simulink model "TPTC_Vehicle_dynamics_pedal2torque_NeglectSOC"  (R2026a)
settings: Solver=ode23tb  StopTime=40
model workspace (MAT data in the model file):
  BattChrgMax = -500000
  BattDischrgMax = 500000
  ChrgLmt_bpt = [1 1 1 1 1 1 1 1 0.7 0.35 0]
  DischrgLmt_bpt = [0 0.35 0.7 1 1 1 1 1 1 1 1]
  SOC_bpt = [0 10 20 30 40 50 60 70 80 90 100]
  motorMaxTorqueNm = [500 500 500 500 500 500 416.666666667 357.142857143 312.5 277.777777778 250 227.272727273 208.333333333 192.307692308 178.571428571 166.666666667]
  motorSpeedRadPs = [0 40 80 120 160 200 240 280 320 360 400 440 480 520 560 600]
values from neighbouring files (symbols this model uses):
  alpha_thr = Simulink.Parameter(300)    [init_MCU_ASR_params_only.m]
  eta_drv = Simulink.Parameter(0.95)    [init_MCU_ASR_params_only.m]
  gear_ratio_F = Simulink.Parameter(10.91)    [init_MCU_ASR_params_only.m]
  gear_ratio_R = Simulink.Parameter(11.62)    [init_MCU_ASR_params_only.m]
  J_axle = Simulink.Parameter(2*I_tire)    [init_MCU_ASR_params_only.m]
  Kd_damp = Simulink.Parameter(0.025)    [init_MCU_ASR_params_only.m]
  R_tire = Simulink.Parameter(r)    [init_MCU_ASR_params_only.m]
  T_active = Simulink.Parameter(15)    [init_MCU_ASR_params_only.m]
  T_damp_lim = Simulink.Parameter(18)    [init_MCU_ASR_params_only.m]
  tau_lpf_damp = Simulink.Parameter(0.060)    [init_MCU_ASR_params_only.m]
  Tlim_down_rate = Simulink.Parameter(2000)    [init_MCU_ASR_params_only.m]
  Tlim_up_rate = Simulink.Parameter(120)    [init_MCU_ASR_params_only.m]
  Tlim_warn_rate = Simulink.Parameter(600)    [init_MCU_ASR_params_only.m]
  Tmax_mot = Simulink.Parameter(Tn_motor)    [init_MCU_ASR_params_only.m]
  Ts_asr = Simulink.Parameter(0.001)    [init_MCU_ASR_params_only.m]
undefined symbols (not defined in the file or in its folder): dspblkCoreblockFVToolHelper, gcbh, gear_ratio
libraries: autolibsharedcoupling x8, simulink x3, autolibshareddiff x2, autolibmappedmotor x2, slpidlib x1, autolibdatasheetbattery x1, sim3dlib x1, sim3dautolib x1, vehdynlibsteering x1
(part 1 of 4)
settings Model: Creator=jchu  LastModifiedBy=woaiw

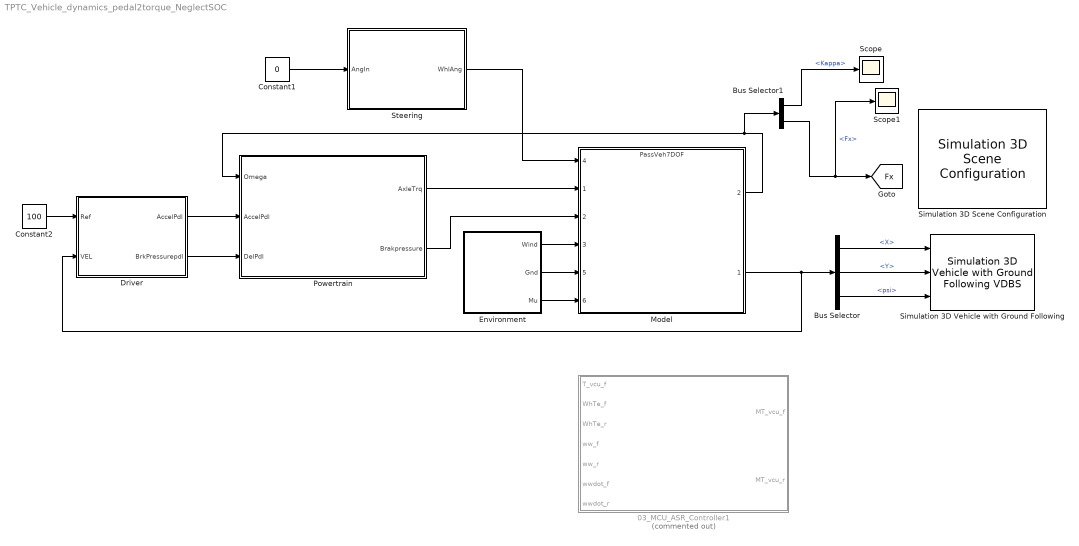
== system TPTC_Vehicle_dynamics_pedal2torque_NeglectSOC ==
  03_MCU_ASR_Controller1 : Subsystem  Commented=on
  Bus Selector : BusSelector  OutputSignals=InertFrm.Cg.Disp.X,InertFrm.Cg.Disp.Y,InertFrm.Cg.Ang.psi
  Bus Selector1 : BusSelector  OutputSignals=TireFrame.Kappa,TireFrame.Fx
  Constant1 : Constant  Value=0
  Constant2 : Constant  Value=100
  Driver : Subsystem
  Environment : Subsystem
      mask Display: disp('Environment')
  Model : ModelReference  ModelNameDialog=PassVeh7DOF.slx  SimulationMode=Normal  ModelReferenceVersion=9.3
      settings: PortSchema="{\"entries\":[{\"content\":{\"sides\":[{\"content\":{\"connectorIds\":[\"In4\",\"In1\",\"In2\",\"In3\",\"In5\",\"In6\"]},\"type\":\"ConnectorPlacement.EquallySpacedRectSide\",\"uuid\":\"e9709a47-3cb3-4a3a-94dc-e137fda36ac7\"},{\"content\":{\"connectorIds\":[\"Out2\",\"Out1\"],\"side\":\"RIGHT\"},\"type\":\"ConnectorPlacement.EquallySpacedRectSide\",\"uuid\":\"17c9465a-c7d2-47f9-932e-b722968c60f5\"},{\"content\":{\"side\":\"TOP\"},\"type\":\"ConnectorPlacement.EquallySpacedRectSide\",\"uuid\":\"38cd0d31-1510-4d7f-a224-4b6e7eb516ec\"}]},\"type\":\"ConnectorPlacement.EquallySpacedConnector\",\"uuid\":\"ef4f9ae8-cb52-4422-b25b-7a352d7601ce\"}],\"packageUris\":[\"http://schema.mathworks.com/mf0/Connector/R2020b\"],\"version\":\"1.0\"}"
  Powertrain : Subsystem
      mask DialogControl ParameterGroupVar Prompt: 参数
      mask Display: image('vdbslibpt.png');
  Scope : Scope
      settings: ActiveDisplayYMinimum=-0.1162629811847193  ActiveDisplayYMaximum=1.0459974821651312  DataLoggingVariableName=ScopeData10
  Scope1 : Scope
      settings: ActiveDisplayYMinimum=-501.51287  ActiveDisplayYMaximum=4500.86669  DataLoggingVariableName=ScopeData9
  Simulation 3D Scene Configuration : sim3dlib/Simulation 3D Scene Configuration  Priority=0  ProjectFormat=Default Scenes  SceneDesc=Straight road  ProjectName=D:\Program Files\MATLAB\R2026a\toolbox\shared\sim3d_projects\automotive_project_windows\UE\WindowsNoEditor\VehicleSimulation.exe  ScenePath=/Game/Maps/HwStrght  EnableOpenDRIVE=off  vehTagList={'Custom';'Scene Origin';'SimulinkVehicle1'}  vehTag=SimulinkVehicle1  AttachedCameraRelativeTranslation=[0 0 0]  FreeCameraDefaultInitialTranslation=[-6, 0, 2]  AttachedCameraRelativeRotation=[0, -15, 0]  FreeCameraDefaultInitialRotation=[0, -15, 0]  ViewpointName=Custom  FreeCameraInitialTranslation=[0, 0, 0]  FreeCameraInitialRotation=[0, 0, 0]  OpVisEn=off  Ts=.02  EnableWindow=on  EnableRemoteAccess=off  SimulationMode=CoSimulation  SimulateUsing=Interpreted execution  EnableAnimationRecording=off  OverrideDefaultRecording=off  AnimationRecordingFileName=sim3dAnimation.mat  AnimationRecordingInterval=[0 inf]  EnableWeather=off  SunAzimuth=90  SunAltitude=40.0  EnableGeospatialSun=off  Latitude=0  Longitude=0  Date=2023-01-01  Time=10:30:00  GeoTimeZone=-5.0  SunDaylightSaving=off  wind=1  clouds=10  EnableVolumetricClouds=off  CloudCoverage=0  CloudAltitude=6  fog=0  rain=0  RaindropsEffect=off  SnowDensity=0  EnableGeospatial=off  TilesetSource=Earth terrain  UseTrueOrigin=off  OriginHeight=200  OriginLatitude=40.744652  OriginLongitude=-73.988864  MapStyle=Aerial  AdditionalAssetIDs=[]  UseAdvancedSunSky=off  SolarTime=11  TimeZone=-5  Day=21  Month=9  Year=2022  UseDaylightSavingTime=on  DSTStartDay=10  DSTStartMonth=3  DSTEndDay=3  DSTEndMonth=11  DSTSwitchHour=2  sensorTag=MainCamera1  sensorId=1  sensorName=MainCamera1  mountLoc=Origin  offsetFlag=off  tmountOffset=[0, 0, 0]  rmountOffset=[0, 0, 0]  HorizontalResolution=1280  VerticalResolution=720  HorizontalFOV=60  mountPoint=[0 0 0]  mountOrientation=[0 0 0]  aMode=2  ID=1  GeoTrigger=Inactive  ViewNameList={'Custom'}  ViewTranslationList={'[0 0 0]'}  ViewRotationList={'[0 0 0]'}
      settings: LibrarySourceBlock=vehdynlibsim3dcore/Simulation 3D Scene Configuration
  Simulation 3D Vehicle with Ground Following : sim3dautolib/Simulation 3D Vehicle with Ground Following VDBS  Priority=-1  PassVehMesh=Muscle car  MeshPath=/MathWorksSimulation/Vehicles/Muscle/Meshes/SK_MuscleCar.SK_MuscleCar  TrackWidth=1.9  WheelBase=3  WheelRadius=0.35  VehColor=Red  CoordinateSystem=Default  InitialPos=[0, 0, 0]  InitialRot=[0, 0, 0]  ActorName=SimulinkVehicle1  VehLightsControl=off  HeadlightColor=[ 1, 1, 1 ]  HighBeamIntensity=100000  LowBeamIntensity=60000  HighBeamConeAngle=1.22  LowBeamConeAngle=1.22  LeftHeadlightOrientation=[ 0, 0 ]  RightHeadlightOrientation=[ 0, 0 ]  BrakelightIntensity=200  ReverselightIntensity=500  SignallightIntensity=500  SignallightPeriod=1  SignalPulseWidth=50  SampleTime=-1  ActorType=SimulinkVehicle  ID=1  aMode=2  ActorTag=SimulinkVehicle1  CoordinateScheme=SAE
      settings: LibrarySourceBlock=vehdynlibsim3d/Simulation 3D Vehicle with Ground Following
  Steering : Subsystem
  tag scope: Fx=global
  wires:
  Bus Selector/2 -> Simulation 3D Vehicle with Ground Following/2  "<Y>"
  Bus Selector/1 -> Simulation 3D Vehicle with Ground Following/1  "<X>"
  Bus Selector/3 -> Simulation 3D Vehicle with Ground Following/3  "<psi>"
  Environment/1(Wind) -> Model/3
  Environment/2(Gnd) -> Model/5
  Environment/3(Mu) -> Model/6
  Constant1/1 -> Steering/1(AngIn)
  Steering/1(WhlAng) -> Model/4
  Model/2 -> Bus Selector1/1, Powertrain/1(Omega)
  Powertrain/2(Brakpressure) -> Model/2
  Constant2/1 -> Driver/1(Ref)
  Model/1 -> Driver/2(VEL), Bus Selector/1
  Driver/1(AccelPdl) -> Powertrain/2(AccelPdl)
  Driver/2(BrkPressurepdl) -> Powertrain/3(DelPdl)
  Powertrain/1(AxleTrq) -> Model/1
  Bus Selector1/1 -> Scope/1  "<Kappa>"
  Bus Selector1/2 -> Scope1/1, [Fx]  "<Fx>"

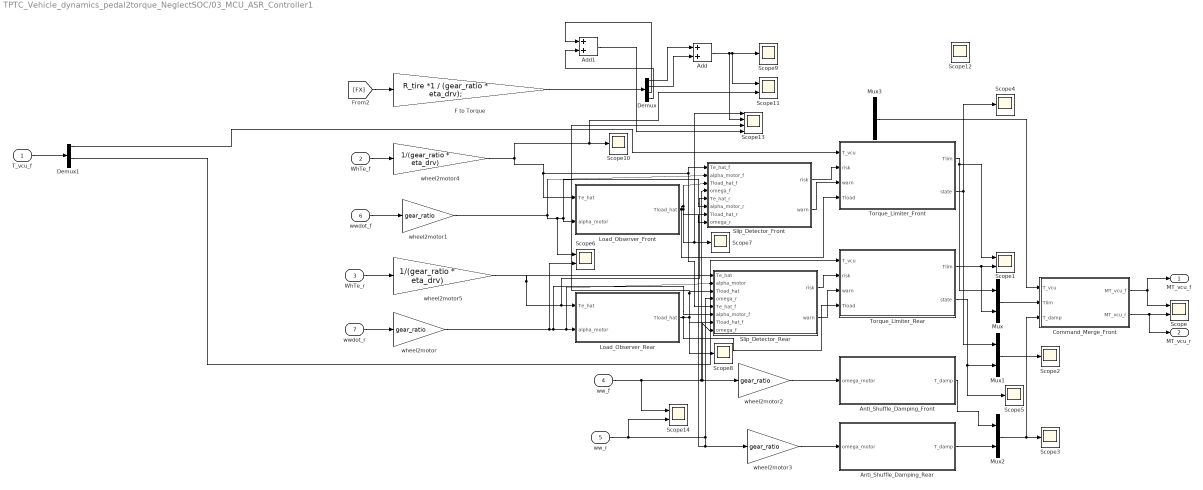
== system TPTC_Vehicle_dynamics_pedal2torque_NeglectSOC/03_MCU_ASR_Controller1 ==
  T_vcu_f : Inport
  WhTe_f : Inport  Port=2
  WhTe_r : Inport  Port=3
  ww_f : Inport  Port=4
  ww_r : Inport  Port=5
  wwdot_f : Inport  Port=6
  wwdot_r : Inport  Port=7
  Add : Sum
  Add1 : Sum
  Anti_Shuffle_Damping_Front : Subsystem
  Anti_Shuffle_Damping_Rear : Subsystem
  Command_Merge_Front : Subsystem
  Demux : Demux
  Demux1 : Demux
  F to Torque : Gain  Gain=R_tire *1 / (gear_ratio * eta_drv);
  Load_Observer_Front : Subsystem
  Load_Observer_Rear : Subsystem
  Mux{,1..3} (4 alike) : Mux  Inputs=2
  Scope{,1,6,11..12,14} (6 alike) : Scope  NumInputPorts=2
      Scope settings: ActiveDisplayYMinimum=-22.2669  ActiveDisplayYMaximum=200.40213  DataLoggingVariableName=ScopeData4
      Scope1 settings: ActiveDisplayYMinimum=-22.33565  ActiveDisplayYMaximum=201.02089  DataLoggingVariableName=ScopeData7
      Scope11 settings: ActiveDisplayYMinimum=-46.74618  ActiveDisplayYMaximum=367.09259  DataLoggingVariableName=ScopeData15
      Scope12 settings: ActiveDisplayYMinimum=-100  ActiveDisplayYMaximum=900  DataLoggingVariableName=ScopeData18
      Scope14 settings: ActiveDisplayYMinimum=23.34376  ActiveDisplayYMaximum=406.47833
      Scope6 settings: ActiveDisplayYMinimum=-2816.65932  ActiveDisplayYMaximum=2610.1461  DataLoggingVariableName=ScopeData11
  Scope{2..5,7..10} (8 alike) : Scope
      Scope10 settings: ActiveDisplayYMinimum=-31.66736  ActiveDisplayYMaximum=285.00624  DataLoggingVariableName=ScopeData12
      Scope2 settings: ActiveDisplayYMinimum=-0.5  ActiveDisplayYMaximum=4.5
      Scope3 settings: ActiveDisplayYMinimum=-15.80377  ActiveDisplayYMaximum=2.40338  DataLoggingVariableName=ScopeData8
      Scope4 settings: ActiveDisplayYMinimum=-0.5  ActiveDisplayYMaximum=4.5  DataLoggingVariableName=ScopeData9
      Scope5 settings: ActiveDisplayYMinimum=-0.5  ActiveDisplayYMaximum=4.5  DataLoggingVariableName=ScopeData10
      Scope7 settings: ActiveDisplayYMinimum=-37.43965  ActiveDisplayYMaximum=336.95687  DataLoggingVariableName=ScopeData4
      Scope8 settings: ActiveDisplayYMinimum=-35.86607  ActiveDisplayYMaximum=322.79459  DataLoggingVariableName=ScopeData5
      Scope9 settings: ActiveDisplayYMinimum=-46.74618  ActiveDisplayYMaximum=367.09259  DataLoggingVariableName=ScopeData6
  Scope13 : Scope  NumInputPorts=4
      settings: ActiveDisplayYMinimum=-50.79662  ActiveDisplayYMaximum=367.54264
  Slip_Detector_Front : Subsystem
  Slip_Detector_Rear : Subsystem
  Torque_Limiter_Front : Subsystem
  Torque_Limiter_Rear : Subsystem
  wheel2motor{,1..3} (4 alike) : Gain  Gain=gear_ratio
  wheel2motor4 : Gain  Gain=1/(gear_ratio * eta_drv)
  wheel2motor5 : Gain  Gain=1/(gear_ratio * eta_drv)
  MT_vcu_f : Outport
  MT_vcu_r : Outport  Port=2
  wires:
  wwdot_f/1 -> wheel2motor1/1
  wwdot_r/1 -> wheel2motor/1
  Load_Observer_Rear/1(Tload_hat) -> Torque_Limiter_Rear/4(Tload), Scope13/3, Slip_Detector_Rear/3(Tload_hat), Scope8/1, Slip_Detector_Rear/7(Tload_hat_f)
  WhTe_r/1 -> wheel2motor5/1
  WhTe_f/1 -> wheel2motor4/1
  wheel2motor/1 -> Slip_Detector_Rear/6(alpha_motor_f), Slip_Detector_Rear/2(alpha_motor), Load_Observer_Rear/2(alpha_motor), Scope6/2
  wheel2motor1/1 -> Scope6/1, Slip_Detector_Front/6(alpha_motor_r), Load_Observer_Front/2(alpha_motor), Slip_Detector_Front/2(alpha_motor_f)
  ww_f/1 -> Scope14/1, wheel2motor2/1, Slip_Detector_Rear/8(omega_f), Slip_Detector_Front/4(omega_f)
  Anti_Shuffle_Damping_Front/1(T_damp) -> Mux2/1
  Slip_Detector_Rear/2(warn) -> Torque_Limiter_Rear/3(warn)
  Slip_Detector_Rear/1(risk) -> Torque_Limiter_Rear/2(risk)
  Slip_Detector_Front/1(risk) -> Torque_Limiter_Front/2(risk)
  Slip_Detector_Front/2(warn) -> Torque_Limiter_Front/3(warn)
  wheel2motor2/1 -> Anti_Shuffle_Damping_Front/1(omega_motor)
  wheel2motor3/1 -> Anti_Shuffle_Damping_Rear/1(omega_motor)
  Mux3/1 -> Command_Merge_Front/1(T_vcu)
  Torque_Limiter_Front/1(Tlim) -> Scope1/1, Mux/1
  Torque_Limiter_Front/2(state) -> Mux1/1, Scope4/1
  Torque_Limiter_Rear/1(Tlim) -> Scope1/2, Mux/2
  Torque_Limiter_Rear/2(state) -> Scope5/1, Mux1/2
  Anti_Shuffle_Damping_Rear/1(T_damp) -> Mux2/2
  Mux/1 -> Command_Merge_Front/2(Tlim)
  Mux1/1 -> Scope2/1
  Mux2/1 -> Scope3/1, Command_Merge_Front/3(T_damp)
  Command_Merge_Front/1(MT_vcu_f) -> MT_vcu_f/1, Scope/1
  Command_Merge_Front/2(MT_vcu_r) -> Scope/2, MT_vcu_r/1
  [FX] -> F to Torque/1
  F to Torque/1 -> Demux/1
  Demux/1 -> Add/1
  Demux/2 -> Add/2
  wheel2motor4/1 -> Slip_Detector_Rear/5(Te_hat_f), Slip_Detector_Front/1(Te_hat_f), Load_Observer_Front/1(Te_hat), Scope11/2, Scope10/1
  wheel2motor5/1 -> Slip_Detector_Front/5(Te_hat_r), Load_Observer_Rear/1(Te_hat), Slip_Detector_Rear/1(Te_hat)
  Demux/3 -> Add1/1
  Demux/4 -> Add1/2
  Load_Observer_Front/1(Tload_hat) -> Scope13/1, Scope7/1, Slip_Detector_Front/7(Tload_hat_r), Slip_Detector_Front/3(Tload_hat_f), Torque_Limiter_Front/4(Tload)
  Add/1 -> Scope13/2, Scope11/1, Scope9/1
  Add1/1 -> Scope13/4
  ww_r/1 -> Scope14/2, wheel2motor3/1, Slip_Detector_Front/8(omega_r), Slip_Detector_Rear/4(omega_r)
  Demux1/1 -> Torque_Limiter_Front/1(T_vcu)
  Demux1/3 -> Torque_Limiter_Rear/1(T_vcu)
  T_vcu_f/1 -> Demux1/1

== system TPTC_Vehicle_dynamics_pedal2torque_NeglectSOC/Driver ==
  Ref : Inport
  VEL : Inport  Port=2
  APPDynamics : TransferFcn  Denominator=[0.75 1]
  Accel : Saturate  UpperLimit=100  LowerLimit=0
  Add : Sum  Inputs=+-
  Brake : Saturate  UpperLimit=0  LowerLimit=-100
  BrakeDynamics : TransferFcn  Denominator=[1 1]
  Bus Selector : BusSelector  OutputSignals=BdyFrm.Cg.Vel.xdot
  Gain : Gain  Gain=1/100
  Gain1 : Gain  Gain=1/100
  MakePositive : Abs  SaturateOnIntegerOverflow=off
  PID Controller : slpidlib/PID Controller  Controller=PI  Form=Parallel  TimeDomain=Continuous-time  UseExternalTs=off  SampleTime=-1  IntegratorMethod=Forward Euler  FilterMethod=Forward Euler  ControllerParametersSource=internal  P=20  I=1  UseKiTs=off  D=0  UseExternalDerivativeSource=off  N=100  UseFilter=on  TunerSelectOption=Transfer Function Based (PID Tuner App)  InitialConditionSource=internal  InitialConditionForIntegrator=0  InitialConditionForFilter=0  DifferentiatorICPrevScaledInput=0  ExternalReset=none  TrackingMode=off  Kt=1  LimitOutput=on  SatLimitsSource=internal  UpperSaturationLimit=100  LowerSaturationLimit=-100  LinearizeAsGain=on  AntiWindupMode=none  Kb=1  LimitIntegrator=off  UpperIntegratorSaturationLimit=inf  LowerIntegratorSaturationLimit=-inf  POutMin=[]  POutMax=[]  IOutMin=[]  IOutMax=[]  DOutMin=[]  DOutMax=[]  NOutMin=[]  NOutMax=[]  SumOutMin=[]  SumOutMax=[]  SaturationOutMin=[]  SaturationOutMax=[]  PParamMin=[]  PParamMax=[]  IParamMin=[]  IParamMax=[]  DParamMin=[]  DParamMax=[]  NParamMin=[]  NParamMax=[]  KbParamMin=[]  KbParamMax=[]  KtParamMin=[]  KtParamMax=[]  KbOutMin=[]  KbOutMax=[]  KtOutMin=[]  KtOutMax=[]  IntegratorOutMin=[]  IntegratorOutMax=[]  FilterOutMin=[]  FilterOutMax=[]  SumI1OutMin=[]  SumI1OutMax=[]  SumI2OutMin=[]  SumI2OutMax=[]  SumI3OutMin=[]  SumI3OutMax=[]  SumI4OutMin=[]  SumI4OutMax=[]  SumDOutMin=[]  SumDOutMax=[]  DifferentiatorOutMin=[]  DifferentiatorOutMax=[]  FilterDiffOutCoefMin=[]  FilterDiffOutCoefMax=[]  ReciprocalOutMin=[]  ReciprocalOutMax=[]  SumDenOutMin=[]  SumDenOutMax=[]  SumNumOutMin=[]  SumNumOutMax=[]  DivideOutMin=[]  DivideOutMax=[]  UdiffTsProdOutMin=[]  UdiffTsProdOutMax=[]  NTsProdOutMin=[]  NTsProdOutMax=[]  UintegralTsProdOutMin=[]  UintegralTsProdOutMax=[]  UngainTsProdOutMin=[]  UngainTsProdOutMax=[]  ClampingZeroOutDataTypeStr=Inherit: Inherit via back propagation  ClampingZeroOutMin=[]  ClampingZeroOutMax=[]  FilterDenConstantOutDataTypeStr=Inherit: Inherit via back propagation  FilterDenConstantOutMin=[]  FilterDenConstantOutMax=[]  PCopyOutDataTypeStr=Inherit: Inherit via back propagation  PCopyOutMin=[]  PCopyOutMax=[]  NCopyOutDataTypeStr=Inherit: Inherit via back propagation  NCopyOutMin=[]  NCopyOutMax=[]  IntegratorContinuousStateAttributes=''  IntegratorStateMustResolveToSignalObject=off  IntegratorRTWStateStorageClass=Auto  FilterContinuousStateAttributes=''  FilterStateMustResolveToSignalObject=off  FilterRTWStateStorageClass=Auto  ParallelPVariant=InternalParameters  IdealPVariant=Disabled  IVariant=InternalParameters  DVariant=Disabled  IntegratorVariant=Continuous  SatVariant=Enabled  AWVariant=Passthrough  PCopyVariant=Disabled  TRVariant=Disabled  FdbkBlocksVariant=Forward  IdealPFdbkVariant=Disabled  SatFdbkVariant=Disabled  DerivativeFilterVariant=Disabled  NVariant=Disabled  NCopyVariant=Disabled_SignalSpec  FilterICVariant=Disabled  IntegratorICVariant=InternalICs  ExternalResetVariant=Disabled  TRSumVariant=Passthrough  SumFdbkVariant=Disabled  SumVariant=Sum_PI  TsampFilterVariant=InternalTs  TsampNgainVariant=Passthrough  TsampIntegralVariant=Disabled_SignalSpec  ExternalSaturationOutDataTypeStr=Inherit: Same as second input  DerivativeSourceVariant=Disabled  PreIntVariant=InternalPreInt
  Scope : Scope
      settings: ActiveDisplayYMinimum=-10.41558  ActiveDisplayYMaximum=93.74018
  AccelPdl : Outport
  BrkPressurepdl : Outport  Port=2
  wires:
  APPDynamics/1 -> Gain/1
  PID Controller/1 -> Accel/1, Brake/1
  MakePositive/1 -> BrakeDynamics/1
  Accel/1 -> APPDynamics/1
  Add/1 -> PID Controller/1
  Brake/1 -> MakePositive/1
  Ref/1 -> Add/1
  BrakeDynamics/1 -> Gain1/1
  Gain/1 -> AccelPdl/1
  Gain1/1 -> BrkPressurepdl/1
  VEL/1 -> Bus Selector/1
  Bus Selector/1 -> Scope/1, Add/2  "<xdot>"

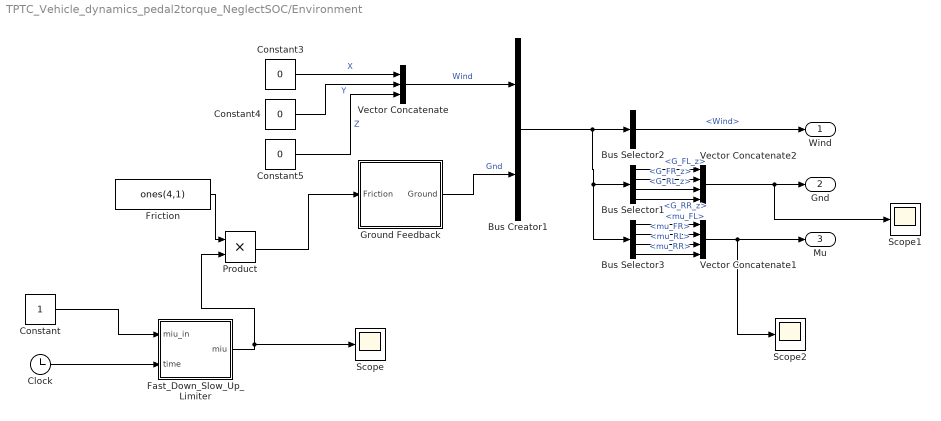
== system TPTC_Vehicle_dynamics_pedal2torque_NeglectSOC/Environment ==
  Bus Creator1 : BusCreator  Inputs=2
  Bus Selector1 : BusSelector  OutputSignals=Gnd.z.G_FL_z,Gnd.z.G_FR_z,Gnd.z.G_RL_z,Gnd.z.G_RR_z
  Bus Selector2 : BusSelector  OutputSignals=Wind
  Bus Selector3 : BusSelector  OutputSignals=Gnd.mu.mu_FL,Gnd.mu.mu_FR,Gnd.mu.mu_RL,Gnd.mu.mu_RR
  Clock : Clock
  Constant : Constant
  Constant3 : Constant  Value=0
  Constant4 : Constant  Value=0
  Constant5 : Constant  Value=0
  Fast_Down_Slow_Up_Limiter : MATLAB Function  TreatAsAtomicUnit=on  SystemSampleTime=Ts_asr
  Friction : Constant  Value=ones(4,1)
  Ground Feedback : Subsystem  Variant=on  VariantControlMode=label  LabelModeActiveChoice=0
  Product : Product
  Scope : Scope
      settings: ActiveDisplayYMinimum=0.2125  ActiveDisplayYMaximum=1.0875  DataLoggingVariableName=ScopeData7
  Scope1 : Scope
      settings: ActiveDisplayYMinimum=-1  ActiveDisplayYMaximum=1  DataLoggingVariableName=ScopeData12
  Scope2 : Scope
      settings: ActiveDisplayYMinimum=0.2125  ActiveDisplayYMaximum=1.0875  DataLoggingVariableName=ScopeData11
  Vector Concatenate : Concatenate  NumInputs=3
  Vector Concatenate1 : Concatenate  NumInputs=4
  Vector Concatenate2 : Concatenate  NumInputs=4
  Wind : Outport
  Gnd : Outport  Port=2
  Mu : Outport  Port=3
  wires:
  Constant5/1 -> Vector Concatenate/3  "Z"
  Vector Concatenate/1 -> Bus Creator1/1  "Wind"
  Constant3/1 -> Vector Concatenate/1  "X"
  Constant4/1 -> Vector Concatenate/2  "Y"
  Ground Feedback/1(Ground) -> Bus Creator1/2  "Gnd"
  Friction/1 -> Product/1
  Bus Selector3/1 -> Vector Concatenate1/1  "<mu_FL>"
  Vector Concatenate1/1 -> Scope2/1, Mu/1
  Bus Selector2/1 -> Wind/1  "<Wind>"
  Vector Concatenate2/1 -> Scope1/1, Gnd/1
  Bus Selector3/3 -> Vector Concatenate1/3  "<mu_RL>"
  Bus Selector3/4 -> Vector Concatenate1/4  "<mu_RR>"
  Bus Selector1/2 -> Vector Concatenate2/2  "<G_FR_z>"
  Bus Creator1/1 -> Bus Selector3/1, Bus Selector1/1, Bus Selector2/1
  Bus Selector3/2 -> Vector Concatenate1/2  "<mu_FR>"
  Bus Selector1/4 -> Vector Concatenate2/4  "<G_RR_z>"
  Bus Selector1/1 -> Vector Concatenate2/1  "<G_FL_z>"
  Bus Selector1/3 -> Vector Concatenate2/3  "<G_RL_z>"
  Product/1 -> Ground Feedback/1(Friction)
  Clock/1 -> Fast_Down_Slow_Up_Limiter/2(time)
  Constant/1 -> Fast_Down_Slow_Up_Limiter/1(miu_in)
  Fast_Down_Slow_Up_Limiter/1(miu) -> Product/2, Scope/1

== system TPTC_Vehicle_dynamics_pedal2torque_NeglectSOC/Powertrain ==
  Omega : Inport
  AccelPdl : Inport  Port=2
  DelPdl : Inport  Port=3
  03_MCU_TPTC_Controller : Subsystem
  Bus Selector : BusSelector  OutputSignals=TireFrame.Omega
  Demux1 : Demux
  Demux2 : Demux  Outputs=2
  Driveline : Subsystem
  ElectricalSystems : Subsystem
  Scope : Scope
      settings: ActiveDisplayYMinimum=-21121.7975  ActiveDisplayYMaximum=190096.17754  DataLoggingVariableName=ScopeData2
  Selector : Selector  InputPortWidth=1  IndexOptions=Index vector (dialog)  Indices=[1 1 1 1]  OutputSizes=1
  Subsystem3 : Subsystem
  VCU : Subsystem
  AxleTrq : Outport
  Brakpressure : Outport  Port=2
  wires:
  ElectricalSystems/2(SOC) -> VCU/3(SOC)
  Subsystem3/1(AxleTrq) -> AxleTrq/1  "AxleTrq"
  AccelPdl/1 -> VCU/4(AccelPdl)
  Omega/1 -> Bus Selector/1
  Bus Selector/1 -> Demux1/1, Subsystem3/1(WhlSpd)  "<Omega>"
  ElectricalSystems/1(MotSpd) -> VCU/1(MotSpd_F)
  VCU/3(BrakePress) -> [BrkP]
  DelPdl/1 -> VCU/5(DelPdl)
  Selector/1 -> Brakpressure/1
  [BrkP] -> Selector/1
  VCU/1(TrqCmd_F) -> Scope/1, 03_MCU_TPTC_Controller/1(T_vcu_F)
  VCU/2(TrqCmd_R) -> 03_MCU_TPTC_Controller/2(T_vcu_R)
  03_MCU_TPTC_Controller/1("T_cmd_f_limited  ") -> ElectricalSystems/1(TrqMCUCmd_F)
  03_MCU_TPTC_Controller/2("T_cmd_r_limited ") -> ElectricalSystems/2(TrqMCUCmd_R)
  Demux1/3 -> 03_MCU_TPTC_Controller/6(omega_m_r)
  Demux1/1 -> 03_MCU_TPTC_Controller/5(omega_m_f)
  Demux2/1 -> 03_MCU_TPTC_Controller/3(Te_f_actual)
  Demux2/2 -> 03_MCU_TPTC_Controller/4(Te_r_actual1)
  ElectricalSystems/3(Mot2Spd) -> VCU/2(MotSpd_R)
  [Te_actual] -> Demux2/1
  connections:
  Subsystem3/LConn1 -- Driveline/RConn1
  ElectricalSystems/RConn1 -- Driveline/LConn1
  Subsystem3/LConn2 -- Driveline/RConn2
  Subsystem3/LConn3 -- Driveline/RConn3
  Subsystem3/LConn4 -- Driveline/RConn4
  ElectricalSystems/RConn2 -- Driveline/LConn2

== system TPTC_Vehicle_dynamics_pedal2torque_NeglectSOC/Steering ==
  AngIn : Inport
  Ground1 : Ground
  Ground2 : Ground
  Kinematic Steering : vehdynlibsteering/Kinematic Steering  StrgType=Rack and pinion  StrgRatioType=Constant  Loc=Front  NrmlFctr=0.01  TrckWdth=1  WhlBase=1.524  Db=0  StrgRng=1.25*pi  StrgAngBpts="[-6.2832   -5.0265   -3.7699   -2.5133   -1.2566         0    1.2566    2.5133    3.7699    5.0265    6.2832]"  StrgRatioTbl=|  StrgRatio=100  PctAckIn=off  PctAck=100  PctAckTbl=ones(1,11)*100  StrgArmLngth=0.1  RckCsLngth=0.5  TieRodLngth=0.248  D=0.2  PnnRadius=0.00085818  PnnRadiusTbl="[0.0055    0.0055    0.0056    0.0057    0.0058    0.0057    0.0057    0.0057    0.0056    0.0055    0.0055]"  RodLngth=0.1  ParaArmLngth=0.9  aMode=2
      | [13.5000   13.3750   13.2500   13.1250   13.0000   13.0000   13.0000   13.1250   13.2500   13.3750   13.5000
      | ]
  Mux : Mux
  WhlAng : Outport
  wires:
  Kinematic Steering/3 -> Mux/2
  Ground1/1 -> Mux/3
  Ground2/1 -> Mux/4
  Kinematic Steering/2 -> Mux/1
  Mux/1 -> WhlAng/1
  AngIn/1 -> Kinematic Steering/1

== system TPTC_Vehicle_dynamics_pedal2torque_NeglectSOC/03_MCU_ASR_Controller1/Anti_Shuffle_Damping_Front ==
  omega_motor : Inport
  Damp_Limit : Saturate  UpperLimit=T_damp_lim  LowerLimit=-T_damp_lim
  HighPass : Sum  Inputs=+-
  LPF_omega : DiscreteTransferFcn  Numerator=[Ts_asr/tau_lpf_damp]  Denominator=[1 -(1-Ts_asr/tau_lpf_damp)]  SampleTime=Ts_asr
  Minus_Kd : Gain  Gain=-Kd_damp
  T_damp : Outport
  wires:
  omega_motor/1 -> LPF_omega/1, HighPass/1
  LPF_omega/1 -> HighPass/2
  HighPass/1 -> Minus_Kd/1
  Minus_Kd/1 -> Damp_Limit/1
  Damp_Limit/1 -> T_damp/1

== system TPTC_Vehicle_dynamics_pedal2torque_NeglectSOC/03_MCU_ASR_Controller1/Anti_Shuffle_Damping_Rear ==
  omega_motor : Inport
  Damp_Limit : Saturate  UpperLimit=T_damp_lim  LowerLimit=-T_damp_lim
  HighPass : Sum  Inputs=+-
  LPF_omega : DiscreteTransferFcn  Numerator=[Ts_asr/tau_lpf_damp]  Denominator=[1 -(1-Ts_asr/tau_lpf_damp)]  SampleTime=Ts_asr
  Minus_Kd : Gain  Gain=-Kd_damp
  T_damp : Outport
  wires:
  omega_motor/1 -> LPF_omega/1, HighPass/1
  LPF_omega/1 -> HighPass/2
  HighPass/1 -> Minus_Kd/1
  Minus_Kd/1 -> Damp_Limit/1
  Damp_Limit/1 -> T_damp/1

== system TPTC_Vehicle_dynamics_pedal2torque_NeglectSOC/03_MCU_ASR_Controller1/Command_Merge_Front ==
  T_vcu : Inport
  Tlim : Inport  Port=2
  T_damp : Inport  Port=3
  Demux1 : Demux  Outputs=2
  Demux2 : Demux  Outputs=2
  Demux3 : Demux  Outputs=2
  Fast_Down_Slow_Up_Limiter : MATLAB Function  TreatAsAtomicUnit=on
  MT_vcu_f : Outport
  MT_vcu_r : Outport  Port=2
  wires:
  Fast_Down_Slow_Up_Limiter/2(T_cmd_r) -> MT_vcu_r/1
  Fast_Down_Slow_Up_Limiter/1(T_cmd_f) -> MT_vcu_f/1
  T_vcu/1 -> Demux1/1
  Demux1/1 -> Fast_Down_Slow_Up_Limiter/1(T_vcu_f)
  Demux1/2 -> Fast_Down_Slow_Up_Limiter/2(T_vcu_r)
  Tlim/1 -> Demux2/1
  Demux2/1 -> Fast_Down_Slow_Up_Limiter/3(Tlim_f)
  Demux2/2 -> Fast_Down_Slow_Up_Limiter/4(Tlim_r)
  T_damp/1 -> Demux3/1
  Demux3/1 -> Fast_Down_Slow_Up_Limiter/5(T_damp_f)
  Demux3/2 -> Fast_Down_Slow_Up_Limiter/6(T_damp_r)

== system TPTC_Vehicle_dynamics_pedal2torque_NeglectSOC/03_MCU_ASR_Controller1/Load_Observer_Front ==
  Te_hat : Inport
  alpha_motor : Inport  Port=2
  J_eq_motor : Gain  Gain=J_axle/(gear_ratio*gear_ratio*eta_drv)
  Saturation_nonnegative : Saturate  UpperLimit=Tmax_mot  LowerLimit=0
  Scope1 : Scope
      settings: ActiveDisplayYMinimum=-88.64455  ActiveDisplayYMaximum=794.81375  DataLoggingVariableName=ScopeData13
  Scope2 : Scope
      settings: ActiveDisplayYMinimum=-299.79825  ActiveDisplayYMaximum=279.9751  DataLoggingVariableName=ScopeData14
  Scope3 : Scope
      settings: ActiveDisplayYMinimum=-4613.8951  ActiveDisplayYMaximum=4308.81674  DataLoggingVariableName=ScopeData16
  Te_minus_Jalpha : Sum  Inputs=+-
  Tload_hat : Outport
  wires:
  alpha_motor/1 -> Scope3/1, J_eq_motor/1
  Te_hat/1 -> Te_minus_Jalpha/1
  J_eq_motor/1 -> Scope2/1, Te_minus_Jalpha/2
  Te_minus_Jalpha/1 -> Scope1/1, Saturation_nonnegative/1
  Saturation_nonnegative/1 -> Tload_hat/1

== system TPTC_Vehicle_dynamics_pedal2torque_NeglectSOC/03_MCU_ASR_Controller1/Load_Observer_Rear ==
  Te_hat : Inport
  alpha_motor : Inport  Port=2
  J_eq_motor : Gain  Gain=J_axle/(gear_ratio*gear_ratio*eta_drv)
  Saturation_nonnegative : Saturate  UpperLimit=Tmax_mot  LowerLimit=0
  Te_minus_Jalpha : Sum  Inputs=+-
  Tload_hat : Outport
  wires:
  alpha_motor/1 -> J_eq_motor/1
  Te_hat/1 -> Te_minus_Jalpha/1
  J_eq_motor/1 -> Te_minus_Jalpha/2
  Te_minus_Jalpha/1 -> Saturation_nonnegative/1
  Saturation_nonnegative/1 -> Tload_hat/1

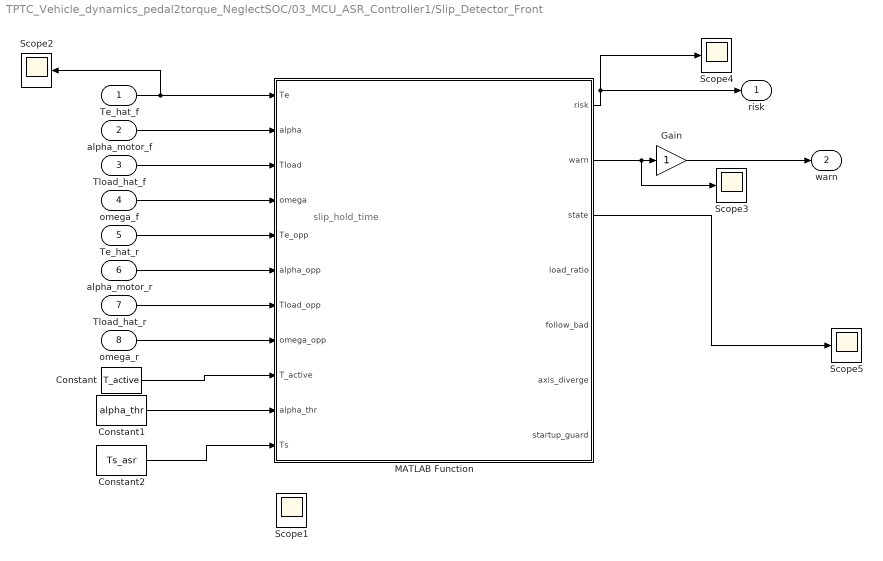
== system TPTC_Vehicle_dynamics_pedal2torque_NeglectSOC/03_MCU_ASR_Controller1/Slip_Detector_Front ==
  note: slip_hold_time
  Te_hat_f : Inport
  alpha_motor_f : Inport  Port=2
  Tload_hat_f : Inport  Port=3
  omega_f : Inport  Port=4
  Te_hat_r : Inport  Port=5
  alpha_motor_r : Inport  Port=6
  Tload_hat_r : Inport  Port=7
  omega_r : Inport  Port=8
  Constant : Constant  Value=T_active
  Constant1 : Constant  Value=alpha_thr
  Constant2 : Constant  Value=Ts_asr
  Gain : Gain
  MATLAB Function : MATLAB Function  TreatAsAtomicUnit=on  SystemSampleTime=Ts_asr
  Scope{1..5} (5 alike) : Scope
      Scope1 settings: ActiveDisplayYMinimum=5  ActiveDisplayYMaximum=25  DataLoggingVariableName=ScopeData10
      Scope2 settings: ActiveDisplayYMinimum=-72.34212  ActiveDisplayYMaximum=651.07911  DataLoggingVariableName=ScopeData11
      Scope3 settings: ActiveDisplayYMinimum=-0.125  ActiveDisplayYMaximum=1.125  DataLoggingVariableName=ScopeData12
      Scope4 settings: ActiveDisplayYMinimum=-0.125  ActiveDisplayYMaximum=1.125  DataLoggingVariableName=ScopeData9
      Scope5 settings: ActiveDisplayYMinimum=-0.25  ActiveDisplayYMaximum=2.25
  risk : Outport
  warn : Outport  Port=2
  wires:
  Tload_hat_f/1 -> MATLAB Function/3(Tload)
  alpha_motor_f/1 -> MATLAB Function/2(alpha)
  Te_hat_f/1 -> Scope2/1, MATLAB Function/1(Te)
  MATLAB Function/1(risk) -> Scope4/1, risk/1
  MATLAB Function/2(warn) -> Scope3/1, Gain/1
  MATLAB Function/3(state) -> Scope5/1
  Gain/1 -> warn/1
  omega_f/1 -> MATLAB Function/4(omega)
  Te_hat_r/1 -> MATLAB Function/5(Te_opp)
  alpha_motor_r/1 -> MATLAB Function/6(alpha_opp)
  Tload_hat_r/1 -> MATLAB Function/7(Tload_opp)
  omega_r/1 -> MATLAB Function/8(omega_opp)
  Constant/1 -> MATLAB Function/9(T_active)
  Constant1/1 -> MATLAB Function/10(alpha_thr)
  Constant2/1 -> MATLAB Function/11(Ts)

== system TPTC_Vehicle_dynamics_pedal2torque_NeglectSOC/03_MCU_ASR_Controller1/Slip_Detector_Rear ==
  Te_hat : Inport
  alpha_motor : Inport  Port=2
  Tload_hat : Inport  Port=3
  omega_r : Inport  Port=4
  Te_hat_f : Inport  Port=5
  alpha_motor_f : Inport  Port=6
  Tload_hat_f : Inport  Port=7
  omega_f : Inport  Port=8
  Constant : Constant  Value=T_active
  Constant1 : Constant  Value=alpha_thr
  Constant2 : Constant  Value=Ts_asr
  MATLAB Function : MATLAB Function  TreatAsAtomicUnit=on  SystemSampleTime=Ts_asr
  Scope : Scope
      settings: ActiveDisplayYMinimum=-0.125  ActiveDisplayYMaximum=1.125  DataLoggingVariableName=ScopeData2
  Scope1 : Scope
      settings: ActiveDisplayYMinimum=-1  ActiveDisplayYMaximum=1  DataLoggingVariableName=ScopeData3
  risk : Outport
  warn : Outport  Port=2
  wires:
  Tload_hat/1 -> MATLAB Function/3(Tload)
  alpha_motor/1 -> MATLAB Function/2(alpha)
  MATLAB Function/2(warn) -> Scope1/1, warn/1
  Te_hat/1 -> MATLAB Function/1(Te)
  MATLAB Function/1(risk) -> Scope/1, risk/1
  omega_r/1 -> MATLAB Function/4(omega)
  Te_hat_f/1 -> MATLAB Function/5(Te_opp)
  alpha_motor_f/1 -> MATLAB Function/6(alpha_opp)
  Tload_hat_f/1 -> MATLAB Function/7(Tload_opp)
  omega_f/1 -> MATLAB Function/8(omega_opp)
  Constant/1 -> MATLAB Function/9(T_active)
  Constant1/1 -> MATLAB Function/10(alpha_thr)
  Constant2/1 -> MATLAB Function/11(Ts)

== system TPTC_Vehicle_dynamics_pedal2torque_NeglectSOC/03_MCU_ASR_Controller1/Torque_Limiter_Front ==
  T_vcu : Inport
  risk : Inport  Port=2
  warn : Inport  Port=3
  Tload : Inport  Port=4
  Fast_Down_Slow_Up_Limiter : MATLAB Function  TreatAsAtomicUnit=on  SystemSampleTime=Ts_asr
  Scope1 : Scope  NumInputPorts=2
      settings: ActiveDisplayYMinimum=-0.125  ActiveDisplayYMaximum=1.125  DataLoggingVariableName=ScopeData4
  Scope14 : Scope  NumInputPorts=2
      settings: ActiveDisplayYMinimum=-100  ActiveDisplayYMaximum=900  DataLoggingVariableName=ScopeData3
  Tlim : Outport
  state : Outport  Port=2
  wires:
  T_vcu/1 -> Scope14/1, Fast_Down_Slow_Up_Limiter/1(T_vcu)
  risk/1 -> Scope1/1, Scope14/2, Fast_Down_Slow_Up_Limiter/2(risk)
  warn/1 -> Scope1/2, Fast_Down_Slow_Up_Limiter/3(warn)
  Fast_Down_Slow_Up_Limiter/1(Tlim) -> Tlim/1
  Fast_Down_Slow_Up_Limiter/2(state) -> state/1
  Tload/1 -> Fast_Down_Slow_Up_Limiter/4(Tload)

== system TPTC_Vehicle_dynamics_pedal2torque_NeglectSOC/03_MCU_ASR_Controller1/Torque_Limiter_Rear ==
  T_vcu : Inport
  risk : Inport  Port=2
  warn : Inport  Port=3
  Tload : Inport  Port=4
  Fast_Down_Slow_Up_Limiter : MATLAB Function  TreatAsAtomicUnit=on  SystemSampleTime=Ts_asr
  Tlim : Outport
  state : Outport  Port=2
  wires:
  T_vcu/1 -> Fast_Down_Slow_Up_Limiter/1(T_vcu)
  risk/1 -> Fast_Down_Slow_Up_Limiter/2(risk)
  warn/1 -> Fast_Down_Slow_Up_Limiter/3(warn)
  Fast_Down_Slow_Up_Limiter/1(Tlim) -> Tlim/1
  Fast_Down_Slow_Up_Limiter/2(state) -> state/1
  Tload/1 -> Fast_Down_Slow_Up_Limiter/4(Tload)

== system TPTC_Vehicle_dynamics_pedal2torque_NeglectSOC/Environment/Ground Feedback ==
  Friction : Inport
  Constant : Subsystem  VariantControl=0
  Ground : Outport  VectorParamsAs1DForOutWhenUnconnected=off

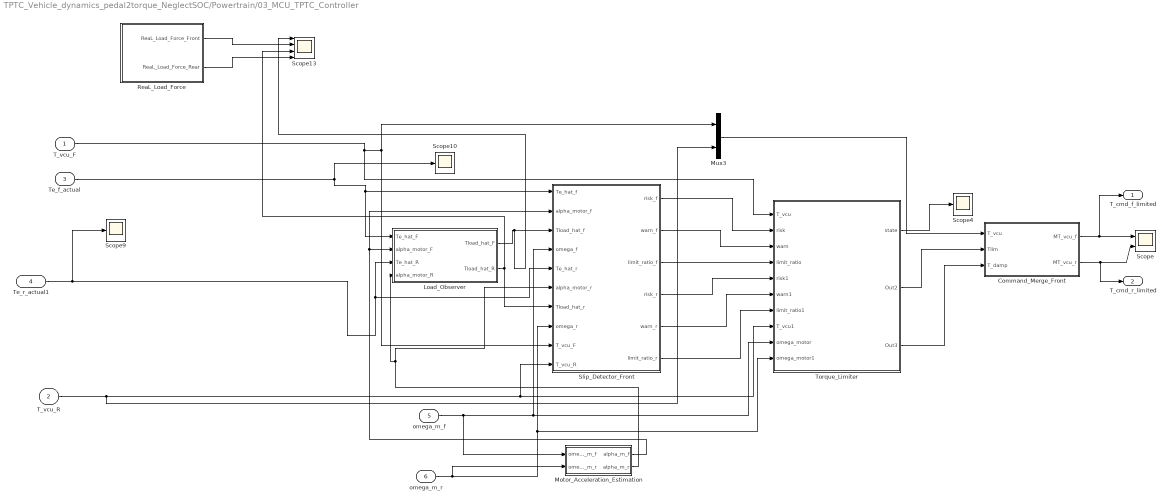
== system TPTC_Vehicle_dynamics_pedal2torque_NeglectSOC/Powertrain/03_MCU_TPTC_Controller ==
  T_vcu_F : Inport
  T_vcu_R : Inport  Port=2
  Te_f_actual : Inport  Port=3
  Te_r_actual1 : Inport  Port=4
  omega_m_f : Inport  Port=5
  omega_m_r : Inport  Port=6
  Command_Merge_Front : Subsystem
  Load_Observer : Subsystem
  Motor_Acceleration_Estimation : Subsystem
  Mux3 : Mux  Inputs=2
  ReaL_Load_Force : Subsystem
  Scope : Scope  NumInputPorts=2
      settings: ActiveDisplayYMinimum=66.18302645192405  ActiveDisplayYMaximum=103.75744150534177  DataLoggingVariableName=ScopeData4
  Scope10 : Scope
      settings: ActiveDisplayYMinimum=-12.5  ActiveDisplayYMaximum=112.5  DataLoggingVariableName=ScopeData12
  Scope13 : Scope  NumInputPorts=4
      settings: ActiveDisplayYMinimum=-30.32591  ActiveDisplayYMaximum=272.21857
  Scope4 : Scope
      settings: ActiveDisplayYMinimum=-0.24999999999999994  ActiveDisplayYMaximum=2.25  DataLoggingVariableName=ScopeData9
  Scope9 : Scope
      settings: ActiveDisplayYMinimum=-12.5  ActiveDisplayYMaximum=112.5  DataLoggingVariableName=ScopeData21
  Slip_Detector_Front : Subsystem
  Torque_Limiter : Subsystem
  "T_cmd_f_limited  " : Outport
  "T_cmd_r_limited " : Outport  Port=2
  wires:
  Motor_Acceleration_Estimation/2(alpha_m_r) -> Slip_Detector_Front/6(alpha_motor_r), Load_Observer/4(alpha_motor_R)
  Motor_Acceleration_Estimation/1(alpha_m_f) -> Slip_Detector_Front/2(alpha_motor_f), Load_Observer/2(alpha_motor_F)
  omega_m_r/1 -> Motor_Acceleration_Estimation/2(omega_m_r), Torque_Limiter/10(omega_motor1), Slip_Detector_Front/8(omega_r)
  Mux3/1 -> Command_Merge_Front/1(T_vcu)
  Command_Merge_Front/1(MT_vcu_f) -> "T_cmd_f_limited  "/1, Scope/1
  Command_Merge_Front/2(MT_vcu_r) -> Scope/2, "T_cmd_r_limited "/1
  Te_f_actual/1 -> Load_Observer/1(Te_hat_F), Slip_Detector_Front/1(Te_hat_f), Scope10/1
  Te_r_actual1/1 -> Scope9/1, Load_Observer/3(Te_hat_R), Slip_Detector_Front/5(Te_hat_r)
  T_vcu_R/1 -> Mux3/2, Torque_Limiter/8(T_vcu1), Slip_Detector_Front/10(T_vcu_R)
  omega_m_f/1 -> Motor_Acceleration_Estimation/1(omega_m_f), Torque_Limiter/9(omega_motor), Slip_Detector_Front/4(omega_f)
  T_vcu_F/1 -> Torque_Limiter/1(T_vcu), Slip_Detector_Front/9(T_vcu_F), Mux3/1
  Load_Observer/1(Tload_hat_F) -> Scope13/1, Slip_Detector_Front/3(Tload_hat_f)
  ReaL_Load_Force/1(ReaL_Load_Force_Front) -> Scope13/2
  ReaL_Load_Force/2(ReaL_Load_Force_Rear) -> Scope13/4
  Load_Observer/2(Tload_hat_R) -> Scope13/3, Slip_Detector_Front/7(Tload_hat_r)
  Slip_Detector_Front/1(risk_f) -> Torque_Limiter/2(risk)
  Slip_Detector_Front/2(warn_f) -> Torque_Limiter/3(warn)
  Slip_Detector_Front/3(limit_ratio_f) -> Torque_Limiter/4(limit_ratio)
  Slip_Detector_Front/4(risk_r) -> Torque_Limiter/5(risk1)
  Slip_Detector_Front/5(warn_r) -> Torque_Limiter/6(warn1)
  Slip_Detector_Front/6(limit_ratio_r) -> Torque_Limiter/7(limit_ratio1)
  Torque_Limiter/1(state) -> Scope4/1
  Torque_Limiter/2(Out2) -> Command_Merge_Front/2(Tlim)
  Torque_Limiter/3(Out3) -> Command_Merge_Front/3(T_damp)

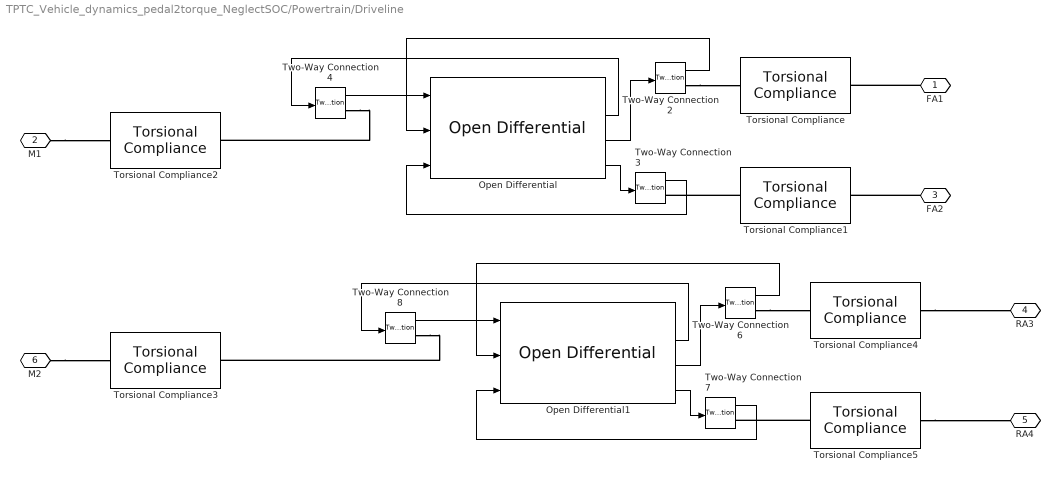
== system TPTC_Vehicle_dynamics_pedal2torque_NeglectSOC/Powertrain/Driveline ==
  Open Differential : autolibshareddiff/Open Differential  DiffEffModelPopup=Constant  InterpMethod=Linear point-slope  extTamb=off  shaftSwitchMask=To the left of center-line  Ndiff=10.91  Jd=.1  bd=1e-3  Jw1=0.019  bw1=1e-3  Jw2=0.019  bw2=1e-3  omegaw1o=0  omegaw2o=0  eta=1  eta_tbl=reshape([0.64 0.76 0.8 0.81 0.83 0.84 0.84 0.56 0.73 0.78 0.8 0.83 0.84 0.84 0.54 0.71 0.77 0.8 0.82 0.84 0.84 0.53 0.71 0.77 0.8 0.83 0.84 0.84 0.51 0.71 0.77 0.8 0.83 0.84 0.85 0.52 0.7 0.77 0.8 0.83 0.84 0.85 0.51 0.71 0.76 0.79 0.83 0.84 0.85 0.5 0.69 0.76 0.79 0.82 0.84 0.85 0.45 0.68 0.75 0.78 0.82 0.84 0.85 0.43 0.67 0.74 0.78 0.81 0.83 0.84 0.38 0.63 0.71 0.75 0.8 0.82 0.83 0.81 0.86 0.88 0.89 0.89 0.89 0.9 0.77 0.85 0.87 0.88 0.89 0.9 0.9 0.72 0.82 0.86 0.87 0.88 0.89 0.9 0.68 0.8 0.84 0.86 0.88 0.89 0.89 0.67 0.8 0.84 0.86 0.88 0.89 0.9 0.67 0.8 0.84 0.86 0.88 0.89 0.9 0.65 0.8 0.84 0.86 0.88 0.89 0.9 0.64 0.79 0.83 0.86 0.88 0.89 0.9 0.63 0.78 0.83 0.86 0.88 0.89 0.9 0.59 0.76 0.82 0.85 0.87 0.89 0.9 0.53 0.73 0.8 0.83 0.86 0.88 0.89], 7, 11, 2)  Trq_bpts=[25, 50, 75, 100, 150, 200, 250]  omega_bpts=[52.4 78.5 105 131 157 183 209 262 314 419 524]  Temp_bpts=[290 358]  Tamb=297.15  maxAbsSpd=5e3  aMode=1
      settings: LibrarySourceBlock=autolibdiff/Open Differential
  Open Differential1 : autolibshareddiff/Open Differential  DiffEffModelPopup=Constant  InterpMethod=Linear point-slope  extTamb=off  shaftSwitchMask=To the left of center-line  Ndiff=11.62  Jd=.1  bd=1e-3  Jw1=0.016  bw1=1e-3  Jw2=0.016  bw2=1e-3  omegaw1o=0  omegaw2o=0  eta=1  eta_tbl=reshape([0.64 0.76 0.8 0.81 0.83 0.84 0.84 0.56 0.73 0.78 0.8 0.83 0.84 0.84 0.54 0.71 0.77 0.8 0.82 0.84 0.84 0.53 0.71 0.77 0.8 0.83 0.84 0.84 0.51 0.71 0.77 0.8 0.83 0.84 0.85 0.52 0.7 0.77 0.8 0.83 0.84 0.85 0.51 0.71 0.76 0.79 0.83 0.84 0.85 0.5 0.69 0.76 0.79 0.82 0.84 0.85 0.45 0.68 0.75 0.78 0.82 0.84 0.85 0.43 0.67 0.74 0.78 0.81 0.83 0.84 0.38 0.63 0.71 0.75 0.8 0.82 0.83 0.81 0.86 0.88 0.89 0.89 0.89 0.9 0.77 0.85 0.87 0.88 0.89 0.9 0.9 0.72 0.82 0.86 0.87 0.88 0.89 0.9 0.68 0.8 0.84 0.86 0.88 0.89 0.89 0.67 0.8 0.84 0.86 0.88 0.89 0.9 0.67 0.8 0.84 0.86 0.88 0.89 0.9 0.65 0.8 0.84 0.86 0.88 0.89 0.9 0.64 0.79 0.83 0.86 0.88 0.89 0.9 0.63 0.78 0.83 0.86 0.88 0.89 0.9 0.59 0.76 0.82 0.85 0.87 0.89 0.9 0.53 0.73 0.8 0.83 0.86 0.88 0.89], 7, 11, 2)  Trq_bpts=[25, 50, 75, 100, 150, 200, 250]  omega_bpts=[52.4 78.5 105 131 157 183 209 262 314 419 524]  Temp_bpts=[290 358]  Tamb=297.15  maxAbsSpd=5e3  aMode=1
      settings: LibrarySourceBlock=autolibdiff/Open Differential
  Torsional Compliance{,1..5} (6 alike) : autolibsharedcoupling/Torsional Compliance  port_config=Two-way connection  extInfo=off  k=1e4  b=1e2  theta_o=0  domega_o=0  omega_c=3000  blkID=0  aMode=1
  Two-Way Connection{2..4,6..8} (6 alike) : TwoWayConnection
  FA1 : PMIOPort  Side=Right
  M1 : PMIOPort  Port=2  Side=Left
  FA2 : PMIOPort  Port=3  Side=Right
  RA3 : PMIOPort  Port=4  Side=Right
  RA4 : PMIOPort  Port=5  Side=Right
  M2 : PMIOPort  Port=6  Side=Left
  wires:
  Two-Way Connection3/1 -> Open Differential/3
  Two-Way Connection2/1 -> Open Differential/2
  Open Differential/4 -> Two-Way Connection3/1
  Open Differential/2 -> Two-Way Connection4/1
  Two-Way Connection4/1 -> Open Differential/1
  Open Differential/3 -> Two-Way Connection2/1
  Two-Way Connection8/1 -> Open Differential1/1
  Open Differential1/3 -> Two-Way Connection6/1
  Two-Way Connection6/1 -> Open Differential1/2
  Two-Way Connection7/1 -> Open Differential1/3
  Open Differential1/2 -> Two-Way Connection8/1
  Open Differential1/4 -> Two-Way Connection7/1
  connections:
  Two-Way Connection2/RConn1 -- Torsional Compliance/LConn1
  M1/RConn1 -- Torsional Compliance2/LConn1
  Two-Way Connection4/RConn1 -- Torsional Compliance2/RConn1
  Torsional Compliance1/LConn1 -- Two-Way Connection3/RConn1
  FA1/RConn1 -- Torsional Compliance/RConn1
  FA2/RConn1 -- Torsional Compliance1/RConn1
  M2/RConn1 -- Torsional Compliance3/LConn1
  Two-Way Connection6/RConn1 -- Torsional Compliance4/LConn1
  Torsional Compliance5/LConn1 -- Two-Way Connection7/RConn1
  Torsional Compliance4/RConn1 -- RA3/RConn1
  Torsional Compliance5/RConn1 -- RA4/RConn1
  Two-Way Connection8/RConn1 -- Torsional Compliance3/RConn1
